simulink model "LQRFirstClosedLoop_Final"  (R2018a)
settings: Solver=VariableStepAuto  StartTime=0.0  StopTime=20  RelTol=1e-3
values from neighbouring files (symbols this model uses):
  A = [0 0 1 0; 0 0 0 1; 0 -m*g/Mc -Kg^2*Km*Kb/(Mc*Rm*r^2) 0; 0 (Mc+m)*g/(Mc*l) Kg^2*Km*Kb/(Mc*Rm*r^2*l) 0]    [InvertedPendulumCode_Final.m]
  B = [0; 0; Km*Kg/(Mc*Rm*r); -Km*Kg/(r*Rm*Mc*l)]    [InvertedPendulumCode_Final.m]
  C = eye(4,4)    [InvertedPendulumCode_Final.m]
  D = zeros(4,1)    [InvertedPendulumCode_Final.m]
  intial_State = [0;0;0;0]    [InvertedPendulumCode_Final.m]
  K = lqr(system_open,Q,R)    [InvertedPendulumCode_Final.m]
  reference_State = [0.2;0;0;0]    [InvertedPendulumCode_Final.m]
settings Model: Creator=jan  LastModifiedBy=DeKon
settings SFSimCC: SimUseLocalCustomCode=on
settings RTWCC: RTWUseLocalCustomCode=on
settings CodeAppCC: StateflowObjectComments=on

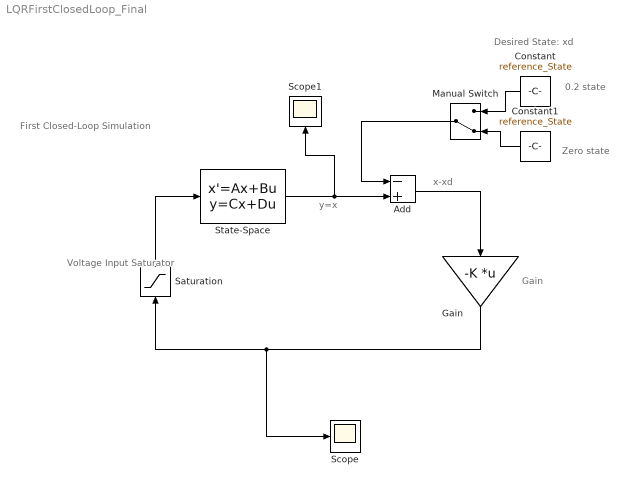
== system LQRFirstClosedLoop_Final ==
  note: 0.2 state
  note: Zero state
  note: Gain
  note: y=x
  note: x-xd
  note: Voltage Input
      | Saturator
  note: First Closed-Loop Simulation
  note: Desired State: xd
  Add : Sum  Inputs=-+
  Constant : Constant  Value=reference_State
  Constant1 : Constant  Value=reference_State
  Gain : Gain  Gain=-K  Multiplication=Matrix(K*u) (u vector)
  Manual Switch : ManualSwitch  CurrentSetting=0
  Saturation : Saturate  UpperLimit=10  LowerLimit=-10
  Scope : Scope
  Scope1 : Scope
  State-Space : StateSpace  A=A  B=B  C=C  D=D  InitialCondition=intial_State
  wires:
  State-Space/1 -> Scope1/1, Add/2
  Add/1 -> Gain/1
  Gain/1 -> Scope/1, Saturation/1
  Saturation/1 -> State-Space/1
  Manual Switch/1 -> Add/1
  Constant/1 -> Manual Switch/1
  Constant1/1 -> Manual Switch/2
